simulink model "AI_Drivers"  (R2020b)
settings: Solver=VariableStepAuto  StartTime=0.0  StopTime=10.0  RelTol=1e-3
undefined symbols (not defined in the file): DiscIntNeverNeededParam
libraries: simulink x7, rllib x2, deeplib x1
(part 1 of 2)
settings Model: Creator=wenka  LastModifiedBy=wenka

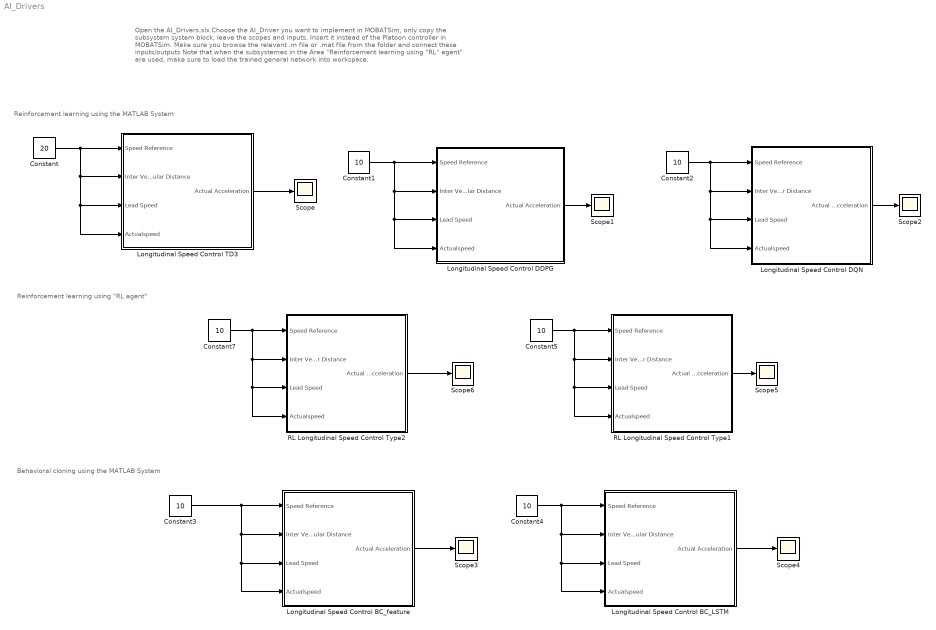
== system AI_Drivers ==
  note: Reinforcement learning using the MATLAB System
  note: Open the AI_Drivers.slx
      | Choose the AI_Driver you want to implement in MOBATSim, only copy the subsystem system block, leave the scopes and inputs.
      | Insert it instead of the Platoon controller in MOBATSim.
      | Make sure you browse the relevant .m file or .mat file from the folder and connect these inputs/outputs
      | Note that when the subsystemes in the Area "Reinforcement learning using "RL" agent" are used, make sure to load the trained general network into workspace.
  note: Behavioral cloning using the MATLAB System
  note: Reinforcement learning using "RL agent"
  Constant : Constant  Value=20  SampleTime=-1
  Constant{1..5,7} (6 alike) : Constant  Value=10  SampleTime=-1
  Longitudinal Speed Control BC_LSTM : Subsystem  mask{Ts=0.01, D_default=25, t_gap=2}
      mask prompts: Ts "Simulink:blkprm_prompts:AllSrcBlksSampleTime"; D_default "Default space"; t_gap "Time gap"
      mask TypeOptions Ts: RL Longitudinal Speed Control/Constant/SampleTime
      mask TypeOptions D_default: Subsystem/Subsystem1/Default Spacing/Value
      mask TypeOptions t_gap: Subsystem/Subsystem1/Time Gap/Value
      mask DialogControl Ts Prompt: Sample time:
  Longitudinal Speed Control BC_feature : Subsystem  mask{Ts=0.01, D_default=25, t_gap=2}
      mask prompts: Ts "Simulink:blkprm_prompts:AllSrcBlksSampleTime"; D_default "Default space"; t_gap "Time gap"
      mask TypeOptions Ts: RL Longitudinal Speed Control/Constant/SampleTime
      mask TypeOptions D_default: Subsystem/Subsystem1/Default Spacing/Value
      mask TypeOptions t_gap: Subsystem/Subsystem1/Time Gap/Value
      mask DialogControl Ts Prompt: Sample time:
  Longitudinal Speed Control DDPG : Subsystem  mask{Ts=0.01, D_default=25, t_gap=1.6}
      mask prompts: Ts "Simulink:blkprm_prompts:AllSrcBlksSampleTime"; D_default "Default space"; t_gap "Time gap"
      mask TypeOptions Ts: RL Longitudinal Speed Control/Constant/SampleTime
      mask TypeOptions D_default: Subsystem/Subsystem1/Default Spacing/Value
      mask TypeOptions t_gap: Subsystem/Subsystem1/Time Gap/Value
      mask DialogControl Ts Prompt: Sample time:
  Longitudinal Speed Control DQN : Subsystem  mask{Ts=0.01, D_default=25, t_gap=1.6}
      mask prompts: Ts "Simulink:blkprm_prompts:AllSrcBlksSampleTime"; D_default "Default space"; t_gap "Time gap"
      mask TypeOptions Ts: RL Longitudinal Speed Control/Constant/SampleTime
      mask TypeOptions D_default: Subsystem/Subsystem1/Default Spacing/Value
      mask TypeOptions t_gap: Subsystem/Subsystem1/Time Gap/Value
      mask DialogControl Ts Prompt: Sample time:
  Longitudinal Speed Control TD3 : Subsystem  mask{Ts=0.01, D_default=25, t_gap=1.6}
      mask prompts: Ts "Simulink:blkprm_prompts:AllSrcBlksSampleTime"; D_default "Default space"; t_gap "Time gap"
      mask TypeOptions Ts: RL Longitudinal Speed Control/Constant/SampleTime
      mask TypeOptions D_default: Subsystem/Subsystem1/Default Spacing/Value
      mask TypeOptions t_gap: Subsystem/Subsystem1/Time Gap/Value
      mask DialogControl Ts Prompt: Sample time:
  RL Longitudinal Speed Control Type1 : Subsystem  mask{Ts=0.01, D_default=25, t_gap=1.6}
      mask prompts: Ts "Simulink:blkprm_prompts:AllSrcBlksSampleTime"; D_default "Default space"; t_gap "Time gap"
      mask TypeOptions Ts: RL Longitudinal Speed Control/Constant/SampleTime
      mask TypeOptions D_default: Subsystem/Subsystem1/Default Spacing/Value
      mask TypeOptions t_gap: Subsystem/Subsystem1/Time Gap/Value
      mask DialogControl Ts Prompt: Sample time:
  RL Longitudinal Speed Control Type2 : Subsystem  mask{Ts=0.01, D_default=25, t_gap=1.6}
      mask prompts: Ts "Simulink:blkprm_prompts:AllSrcBlksSampleTime"; D_default "Default space"; t_gap "Time gap"
      mask TypeOptions Ts: RL Longitudinal Speed Control/Constant/SampleTime
      mask TypeOptions D_default: Subsystem/Subsystem1/Default Spacing/Value
      mask TypeOptions t_gap: Subsystem/Subsystem1/Time Gap/Value
      mask DialogControl Ts Prompt: Sample time:
  Scope{,1..6} (7 alike) : Scope
  wires:
  Constant/1 -> Longitudinal Speed Control TD3/3(Lead Speed), Longitudinal Speed Control TD3/4(Actualspeed), Longitudinal Speed Control TD3/2(Inter Vehicular Distance), Longitudinal Speed Control TD3/1(Speed Reference)
  Constant1/1 -> Longitudinal Speed Control DDPG/4(Actualspeed), Longitudinal Speed Control DDPG/3(Lead Speed), Longitudinal Speed Control DDPG/2(Inter Vehicular Distance), Longitudinal Speed Control DDPG/1(Speed Reference)
  Longitudinal Speed Control TD3/1(Actual Acceleration) -> Scope/1
  Longitudinal Speed Control DDPG/1(Actual Acceleration) -> Scope1/1
  Constant2/1 -> Longitudinal Speed Control DQN/3(Lead Speed), Longitudinal Speed Control DQN/4(Actualspeed), Longitudinal Speed Control DQN/2(Inter Vehicular Distance), Longitudinal Speed Control DQN/1(Speed Reference)
  Longitudinal Speed Control DQN/1(Actual Acceleration) -> Scope2/1
  Constant3/1 -> Longitudinal Speed Control BC_feature/4(Actualspeed), Longitudinal Speed Control BC_feature/3(Lead Speed), Longitudinal Speed Control BC_feature/2(Inter Vehicular Distance), Longitudinal Speed Control BC_feature/1(Speed Reference)
  Longitudinal Speed Control BC_feature/1(Actual Acceleration) -> Scope3/1
  Constant4/1 -> Longitudinal Speed Control BC_LSTM/2(Inter Vehicular Distance), Longitudinal Speed Control BC_LSTM/3(Lead Speed), Longitudinal Speed Control BC_LSTM/4(Actualspeed), Longitudinal Speed Control BC_LSTM/1(Speed Reference)
  Longitudinal Speed Control BC_LSTM/1(Actual Acceleration) -> Scope4/1
  Constant5/1 -> RL Longitudinal Speed Control Type1/1(Speed Reference), RL Longitudinal Speed Control Type1/2(Inter Vehicular Distance), RL Longitudinal Speed Control Type1/4(Actualspeed), RL Longitudinal Speed Control Type1/3(Lead Speed)
  RL Longitudinal Speed Control Type1/1(Actual Acceleration) -> Scope5/1
  Constant7/1 -> RL Longitudinal Speed Control Type2/1(Speed Reference), RL Longitudinal Speed Control Type2/2(Inter Vehicular Distance), RL Longitudinal Speed Control Type2/3(Lead Speed), RL Longitudinal Speed Control Type2/4(Actualspeed)
  RL Longitudinal Speed Control Type2/1(Actual Acceleration) -> Scope6/1

== system AI_Drivers/Longitudinal Speed Control BC_LSTM ==
  note: The block processes the states, rewards and status for training the agent
  note: Output
  note: Reference speed
  note: Speed of the
      | lead vehicle
  note: Distance to the
      | lead vehicle
  note: Input
  note: Actual speed
  Speed Reference : Inport
  Inter Vehicular Distance : Inport  Port=2
  Lead Speed : Inport  Port=3
  Actualspeed : Inport  Port=4
  LSTM_prediction : Subsystem
  Signal Processing for ACC : Subsystem
  Actual Acceleration : Outport  VectorParamsAs1DForOutWhenUnconnected=off
  wires:
  Lead Speed/1 -> Signal Processing for ACC/3(v_lead)
  LSTM_prediction/1(Predicted Acc) -> Actual Acceleration/1
  Speed Reference/1 -> Signal Processing for ACC/2(v_ref)
  Actualspeed/1 -> Signal Processing for ACC/1(v_ego)
  Inter Vehicular Distance/1 -> Signal Processing for ACC/4(d_rel)
  Signal Processing for ACC/1(obs) -> LSTM_prediction/1("dataTest ")

== system AI_Drivers/Longitudinal Speed Control BC_feature ==
  note: The block processes the states, rewards and status for training the agent
  note: Output
  note: Reference speed
  note: Speed of the
      | lead vehicle
  note: Distance to the
      | lead vehicle
  note: Input
  note: Actual speed
  Speed Reference : Inport
  Inter Vehicular Distance : Inport  Port=2
  Lead Speed : Inport  Port=3
  Actualspeed : Inport  Port=4
  MATLAB System : MATLABSystem  System=BC_feature  SimulateUsing=Interpreted execution
      mask Type: BC_feature
      mask Display:
      | disp('BC_feature');
      | port_label('input',1,'DataInput');
      | port_label('output',1,'predictedData');
  Signal Processing for ACC : Subsystem
  Actual Acceleration : Outport  VectorParamsAs1DForOutWhenUnconnected=off
  wires:
  Lead Speed/1 -> Signal Processing for ACC/3(v_lead)
  MATLAB System/1 -> Actual Acceleration/1  "Acc"
  Speed Reference/1 -> Signal Processing for ACC/2(v_ref)
  Actualspeed/1 -> Signal Processing for ACC/1(v_ego)
  Inter Vehicular Distance/1 -> Signal Processing for ACC/4(d_rel)
  Signal Processing for ACC/1(obs) -> MATLAB System/1

== system AI_Drivers/Longitudinal Speed Control DDPG ==
  note: The block processes the states, rewards and status for training the agent
  note: Output
  note: Reference speed
  note: Speed of the
      | lead vehicle
  note: Distance to the
      | lead vehicle
  note: Input
  note: Actual speed
  Speed Reference : Inport
  Inter Vehicular Distance : Inport  Port=2
  Lead Speed : Inport  Port=3
  Actualspeed : Inport  Port=4
  Data Type Conversion : DataTypeConversion  OutDataTypeStr=double
  MATLAB System : MATLABSystem  System=DDPG  SimulateUsing=Interpreted execution
      mask Type: DDPG
      mask Display:
      | disp('DDPG');
      | port_label('input',1,'Obs');
      | port_label('output',1,'predictedAcc');
  Signal Processing for ACC : Subsystem
  Actual Acceleration : Outport  VectorParamsAs1DForOutWhenUnconnected=off
  wires:
  Lead Speed/1 -> Signal Processing for ACC/3(v_lead)
  Speed Reference/1 -> Signal Processing for ACC/2(v_ref)
  Actualspeed/1 -> Signal Processing for ACC/1(v_ego)
  Inter Vehicular Distance/1 -> Signal Processing for ACC/4(d_rel)
  Signal Processing for ACC/1(obs) -> MATLAB System/1
  Data Type Conversion/1 -> Actual Acceleration/1
  MATLAB System/1 -> Data Type Conversion/1  "Acc"

== system AI_Drivers/Longitudinal Speed Control DQN ==
  note: Reference speed
  note: The block processes observations for training the agent
  note: Distance to the
      | lead vehicle
  note: Input
  note: Actual speed
  note: Speed of the
      | lead vehicle
  note: Output
  Speed Reference : Inport
  Inter Vehicular Distance : Inport  Port=2
  Lead Speed : Inport  Port=3
  Actualspeed : Inport  Port=4
  MATLAB System : MATLABSystem  System=DQN  SimulateUsing=Interpreted execution
      mask Type: DQN
      mask Display:
      | disp('DQN');
      | port_label('input',1,'Obs');
      | port_label('input',2,'Action');
      | port_label('output',1,'predictedAcc');
  Signal Processing for ACC : Subsystem
  Unit Delay : UnitDelay  InitialCondition=0.01  SampleTime=Ts  HasFrameUpgradeWarning=on
  Actual Acceleration : Outport  VectorParamsAs1DForOutWhenUnconnected=off
  wires:
  Inter Vehicular Distance/1 -> Signal Processing for ACC/4(d_rel)
  Actualspeed/1 -> Signal Processing for ACC/1(v_ego)
  Speed Reference/1 -> Signal Processing for ACC/2(v_ref)
  Lead Speed/1 -> Signal Processing for ACC/3(v_lead)
  MATLAB System/1 -> Unit Delay/1, Actual Acceleration/1
  Unit Delay/1 -> MATLAB System/2
  Signal Processing for ACC/1(obs) -> MATLAB System/1

== system AI_Drivers/Longitudinal Speed Control TD3 ==
  note: The block processes the states, rewards and status for training the agent
  note: Output
  note: Reference speed
  note: Speed of the
      | lead vehicle
  note: Distance to the
      | lead vehicle
  note: Input
  note: Actual speed
  Speed Reference : Inport
  Inter Vehicular Distance : Inport  Port=2
  Lead Speed : Inport  Port=3
  Actualspeed : Inport  Port=4
  MATLAB System : MATLABSystem  System=TD3  SimulateUsing=Interpreted execution
      mask Type: TD3
      mask Display:
      | disp('TD3');
      | port_label('input',1,'Obs');
      | port_label('output',1,'predictedAcc');
  Signal Processing for ACC : Subsystem
  Actual Acceleration : Outport  VectorParamsAs1DForOutWhenUnconnected=off
  wires:
  Lead Speed/1 -> Signal Processing for ACC/3(v_lead)
  MATLAB System/1 -> Actual Acceleration/1  "Acc"
  Speed Reference/1 -> Signal Processing for ACC/2(v_ref)
  Actualspeed/1 -> Signal Processing for ACC/1(v_ego)
  Inter Vehicular Distance/1 -> Signal Processing for ACC/4(d_rel)
  Signal Processing for ACC/1(obs) -> MATLAB System/1

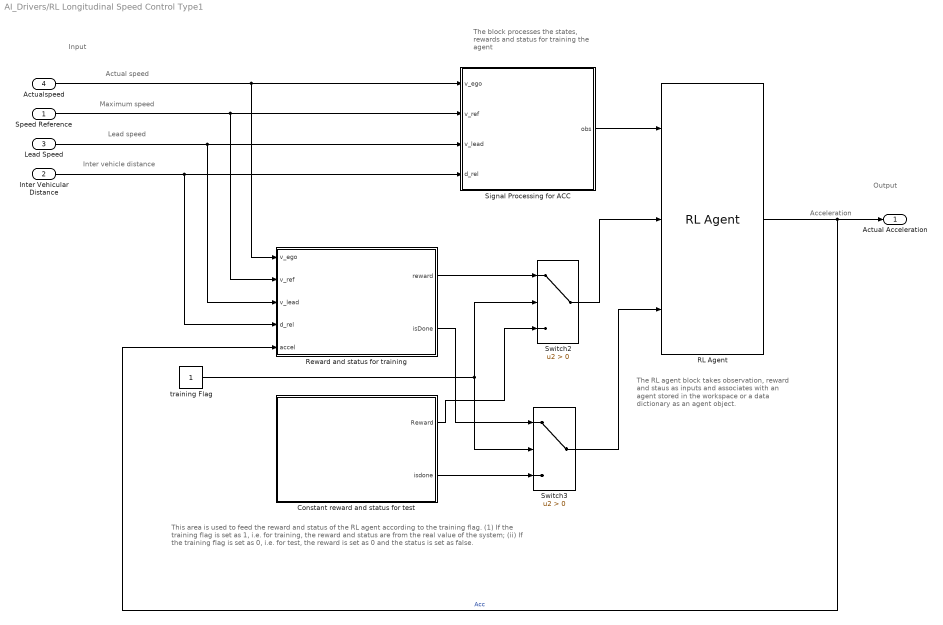
== system AI_Drivers/RL Longitudinal Speed Control Type1 ==
  note: Actual speed
  note: Acceleration
  note: Input
  note: Inter vehicle distance
  note: Lead speed
  note: Output
  note: The RL agent block takes observation, reward and staus as inputs and associates with an agent stored in the workspace or a data dictionary as an agent object.
  note: The block processes the states, rewards and status for training the agent
  note: Maximum speed
  note: This area is used to feed the reward and status of the RL agent according to the training flag.
      | (1) If the training flag is set as 1, i.e. for training, the reward and status are from the real value of the system;
      | (ii) If the training flag is set as 0, i.e. for test, the reward is set as 0 and the status is set as false.
  Speed Reference : Inport
  Inter Vehicular Distance : Inport  Port=2
  Lead Speed : Inport  Port=3
  Actualspeed : Inport  Port=4
  Constant reward and status for test : Subsystem
  RL Agent : rllib/RL Agent  Agent=agent  ProvideReward=on  ProvideIsDone=on  ProvideCumRwd=off  TreatAsDirectFeedthrough=on  CollectLoggedSignals=on  CollectModelStates=on
  Reward and status for training : Subsystem
  Signal Processing for ACC : Subsystem
  Switch2 : Switch  Criteria=u2 > Threshold
  Switch3 : Switch  Criteria=u2 > Threshold
  training Flag : Constant
  Actual Acceleration : Outport  VectorParamsAs1DForOutWhenUnconnected=off
  wires:
  Signal Processing for ACC/1(obs) -> RL Agent/1
  Actualspeed/1 -> Reward and status for training/1(v_ego), Signal Processing for ACC/1(v_ego)
  Speed Reference/1 -> Reward and status for training/2(v_ref), Signal Processing for ACC/2(v_ref)
  Lead Speed/1 -> Reward and status for training/3(v_lead), Signal Processing for ACC/3(v_lead)
  Inter Vehicular Distance/1 -> Reward and status for training/4(d_rel), Signal Processing for ACC/4(d_rel)
  Constant reward and status for test/2(isdone) -> Switch3/3
  training Flag/1 -> Switch2/2, Switch3/2
  Reward and status for training/1(reward) -> Switch2/1
  RL Agent/1 -> Reward and status for training/5(accel), Actual Acceleration/1  "Acc"
  Reward and status for training/2(isDone) -> Switch3/1
  Switch3/1 -> RL Agent/3
  Switch2/1 -> RL Agent/2
  Constant reward and status for test/1(Reward) -> Switch2/3

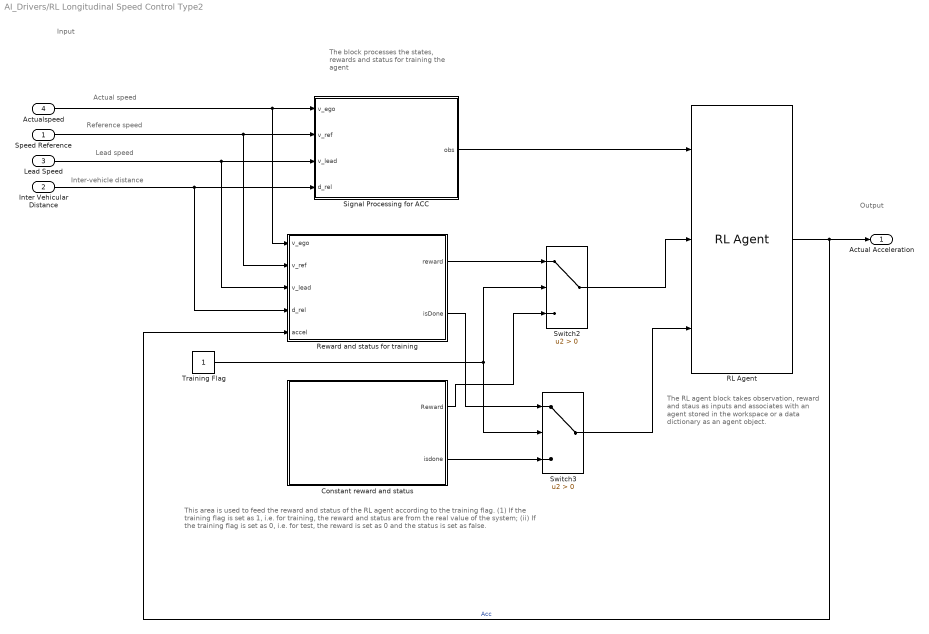
== system AI_Drivers/RL Longitudinal Speed Control Type2 ==
  note: Actual speed
  note: Input
  note: Reference speed
  note: Lead speed
  note: Output
  note: The block processes the states, rewards and status for training the agent
  note: The RL agent block takes observation, reward and staus as inputs and associates with an agent stored in the workspace or a data dictionary as an agent object.
  note: This area is used to feed the reward and status of the RL agent according to the training flag.
      | (1) If the training flag is set as 1, i.e. for training, the reward and status are from the real value of the system;
      | (ii) If the training flag is set as 0, i.e. for test, the reward is set as 0 and the status is set as false.
  note: Inter-vehicle distance
  Speed Reference : Inport
  Inter Vehicular Distance : Inport  Port=2
  Lead Speed : Inport  Port=3
  Actualspeed : Inport  Port=4
  Constant reward and status : Subsystem
  RL Agent : rllib/RL Agent  Agent=agent  ProvideReward=on  ProvideIsDone=on  ProvideCumRwd=off  TreatAsDirectFeedthrough=on  CollectLoggedSignals=on  CollectModelStates=on
  Reward and status for training : Subsystem
  Signal Processing for ACC : Subsystem
  Switch2 : Switch  Criteria=u2 > Threshold
  Switch3 : Switch  Criteria=u2 > Threshold
  Training Flag : Constant
  Actual Acceleration : Outport  VectorParamsAs1DForOutWhenUnconnected=off
  wires:
  Lead Speed/1 -> Reward and status for training/3(v_lead), Signal Processing for ACC/3(v_lead)
  Actualspeed/1 -> Reward and status for training/1(v_ego), Signal Processing for ACC/1(v_ego)
  Training Flag/1 -> Switch2/2, Switch3/2
  Constant reward and status/2(isdone) -> Switch3/3
  Reward and status for training/1(reward) -> Switch2/1
  Signal Processing for ACC/1(obs) -> RL Agent/1
  Reward and status for training/2(isDone) -> Switch3/1
  Switch3/1 -> RL Agent/3
  Switch2/1 -> RL Agent/2
  Constant reward and status/1(Reward) -> Switch2/3
  RL Agent/1 -> Reward and status for training/5(accel), Actual Acceleration/1  "Acc"
  Inter Vehicular Distance/1 -> Reward and status for training/4(d_rel), Signal Processing for ACC/4(d_rel)
  Speed Reference/1 -> Reward and status for training/2(v_ref), Signal Processing for ACC/2(v_ref)

== system AI_Drivers/Longitudinal Speed Control BC_LSTM/LSTM_prediction ==
  note: The Predict block predicts responses for the data at the input by using the trained network specified through the block parameter.
  note: This block normalizes the training predictors to have zero mean and unit variance
  "dataTest " : Inport
  MATLAB Function : MATLAB Function  TreatAsAtomicUnit=on  SystemSampleTime=Ts
  Mu File : FromFile  FileName=LSTM_mu.mat  SampleTime=0
  Predictor : deeplib/Predict  Network=Network from MAT-file  NetworkFunction=squeezenet  NetworkFilePath=C:\Users\wenka\OneDrive\Documents\GitHub\MOBATSim\AI_Drivers\BC_LSTM\BiLSTMnet.mat  MiniBatchSize=1  InputDataFormats={ '', '' }  Predictions=on  Activations={}  ForceInterpretedSim=off  EnableDLNetwork=off
      settings: SourceProductBaseCode=NN
  Sig File : FromFile  FileName=LSTM_sig.mat  SampleTime=0
  Predicted Acc : Outport
  wires:
  Sig File/1 -> MATLAB Function/3(sigFile)
  Predictor/1 -> Predicted Acc/1
  MATLAB Function/1(dataTest) -> Predictor/1
  "dataTest "/1 -> MATLAB Function/1("dataTest ")
  Mu File/1 -> MATLAB Function/2(muFile)

== system AI_Drivers/Longitudinal Speed Control BC_LSTM/Signal Processing for ACC ==
  note: observation
  note: Input
  note: Relative distance
  note: Ego speed
  note: Lead speed
  note: Maximum speed
  note: This subsystem calculates
      | the safe distance
  note: Output
  note: This subsystem calculates
      | the error between the ego
      | speed and target speed
  note: Relative distance
  note: Ego speed
  note: Speed error
  note: Lead speed
  note: Safe distance
  v_ego : Inport
  v_ref : Inport  Port=2
  v_lead : Inport  Port=3
  d_rel : Inport  Port=4
  Calculates speed error : Subsystem
  Mux : Mux  Inputs=5
  Safe distance : Subsystem
  obs : Outport  VectorParamsAs1DForOutWhenUnconnected=off
  wires:
  v_ego/1 -> Mux/5, Calculates speed error/3(v_ego), Safe distance/2(v_ego)
  d_rel/1 -> Mux/2, Safe distance/1(relative distance)
  Mux/1 -> obs/1
  Safe distance/2(Distance error) -> Calculates speed error/2(d_err)
  v_lead/1 -> Calculates speed error/1(v_lead), Mux/1
  v_ref/1 -> Calculates speed error/4(v_set)
  Safe distance/1(Safe distance) -> Mux/3
  Calculates speed error/1(v_err) -> Mux/4

== system AI_Drivers/Longitudinal Speed Control BC_feature/Signal Processing for ACC ==
  note: observation
  note: Input
  note: Relative distance
  note: Ego speed
  note: Lead speed
  note: Maximum speed
  note: This subsystem calculates
      | the safe distance
  note: Output
  note: This subsystem calculates
      | the error between the ego
      | speed and target speed
  note: Relative distance
  note: Ego speed
  note: Speed error
  note: Lead speed
  note: Safe distance
  v_ego : Inport
  v_ref : Inport  Port=2
  v_lead : Inport  Port=3
  d_rel : Inport  Port=4
  Calculates speed error : Subsystem
  Mux : Mux  Inputs=5
  Safe distance : Subsystem
  obs : Outport  VectorParamsAs1DForOutWhenUnconnected=off
  wires:
  v_ego/1 -> Mux/5, Calculates speed error/3(v_ego), Safe distance/2(v_ego)
  d_rel/1 -> Mux/2, Safe distance/1(relative distance)
  Mux/1 -> obs/1
  Safe distance/2(Distance error) -> Calculates speed error/2(d_err)
  v_lead/1 -> Calculates speed error/1(v_lead), Mux/1
  v_ref/1 -> Calculates speed error/4(v_set)
  Safe distance/1(Safe distance) -> Mux/3
  Calculates speed error/1(v_err) -> Mux/4

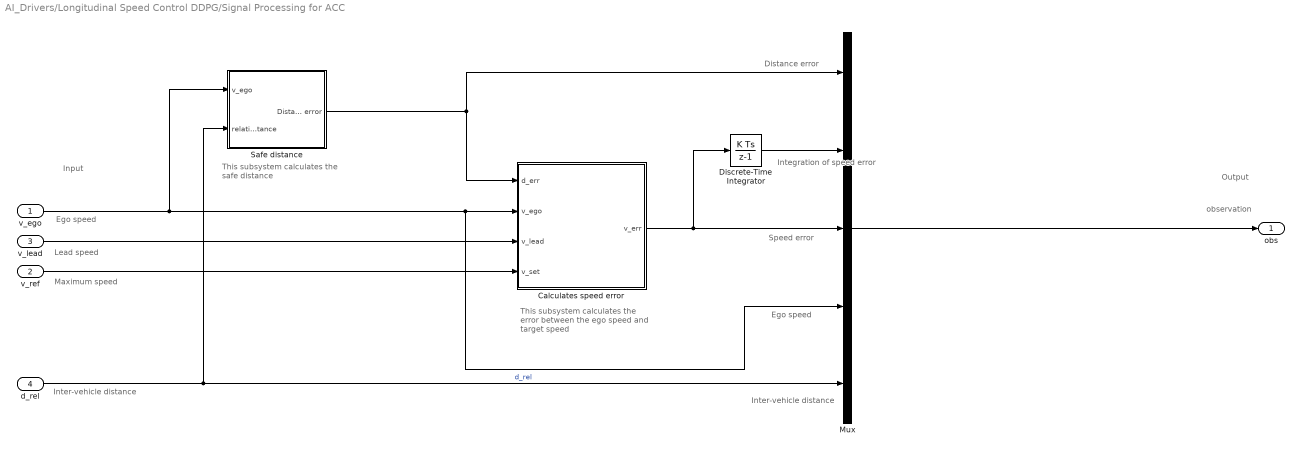
== system AI_Drivers/Longitudinal Speed Control DDPG/Signal Processing for ACC ==
  note: Distance error
  note: observation
  note: Input
  note: Inter-vehicle distance
  note: Ego speed
  note: Lead speed
  note: Maximum speed
  note: This subsystem calculates
      | the safe distance
  note: Output
  note: This subsystem calculates
      | the error between the ego
      | speed and target speed
  note: Inter-vehicle distance
  note: Ego speed
  note: Speed error
  note: Integration of
      | speed error
  v_ego : Inport
  v_ref : Inport  Port=2
  v_lead : Inport  Port=3
  d_rel : Inport  Port=4
  Calculates speed error : Subsystem
  Discrete-Time Integrator : DiscreteIntegrator  SampleTime=-1  ICPrevOutput=DiscIntNeverNeededParam  ICPrevScaledInput=DiscIntNeverNeededParam
  Mux : Mux  Inputs=5
  Safe distance : Subsystem
  obs : Outport  VectorParamsAs1DForOutWhenUnconnected=off
  wires:
  v_ego/1 -> Safe distance/1(v_ego), Calculates speed error/2(v_ego), Mux/4
  d_rel/1 -> Mux/5, Safe distance/2(relative distance)  "d_rel"
  Discrete-Time Integrator/1 -> Mux/2
  Safe distance/1(Distance error) -> Calculates speed error/1(d_err), Mux/1
  Calculates speed error/1(v_err) -> Discrete-Time Integrator/1, Mux/3
  v_lead/1 -> Calculates speed error/3(v_lead)
  v_ref/1 -> Calculates speed error/4(v_set)
  Mux/1 -> obs/1

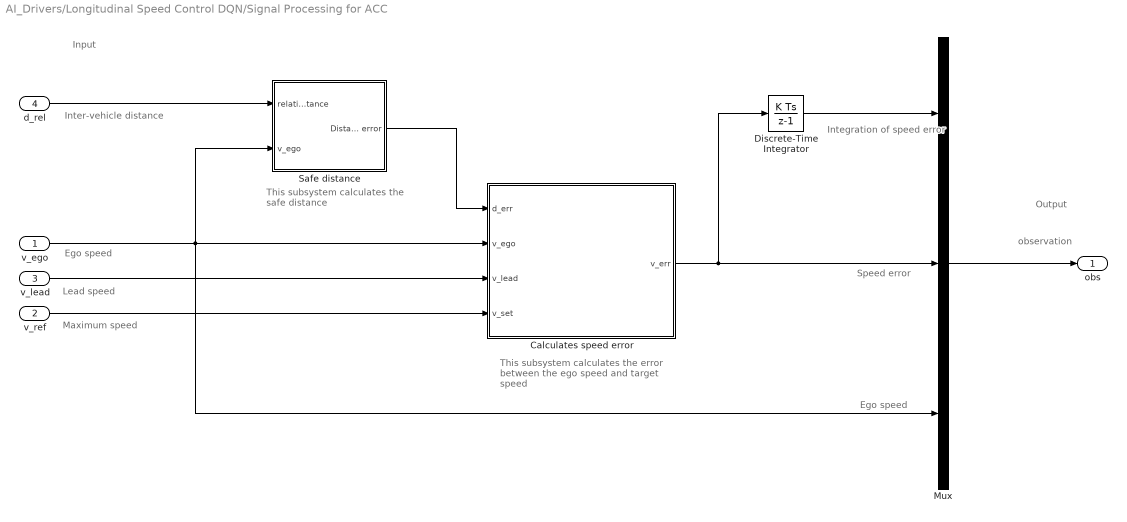
== system AI_Drivers/Longitudinal Speed Control DQN/Signal Processing for ACC ==
  note: observation
  note: Input
  note: Inter-vehicle distance
  note: Ego speed
  note: Lead speed
  note: Maximum speed
  note: This subsystem calculates
      | the safe distance
  note: Output
  note: This subsystem calculates
      | the error between the ego
      | speed and target speed
  note: Ego speed
  note: Speed error
  note: Integration of
      | speed error
  v_ego : Inport
  v_ref : Inport  Port=2
  v_lead : Inport  Port=3
  d_rel : Inport  Port=4
  Calculates speed error : Subsystem
  Discrete-Time Integrator : DiscreteIntegrator  SampleTime=-1  ICPrevOutput=DiscIntNeverNeededParam  ICPrevScaledInput=DiscIntNeverNeededParam
  Mux : Mux  Inputs=3
  Safe distance : Subsystem
  obs : Outport  VectorParamsAs1DForOutWhenUnconnected=off
  wires:
  v_ego/1 -> Mux/3, Safe distance/2(v_ego), Calculates speed error/2(v_ego)
  d_rel/1 -> Safe distance/1(relative distance)
  Safe distance/1(Distance error) -> Calculates speed error/1(d_err)
  Calculates speed error/1(v_err) -> Discrete-Time Integrator/1, Mux/2
  v_lead/1 -> Calculates speed error/3(v_lead)
  v_ref/1 -> Calculates speed error/4(v_set)
  Mux/1 -> obs/1
  Discrete-Time Integrator/1 -> Mux/1

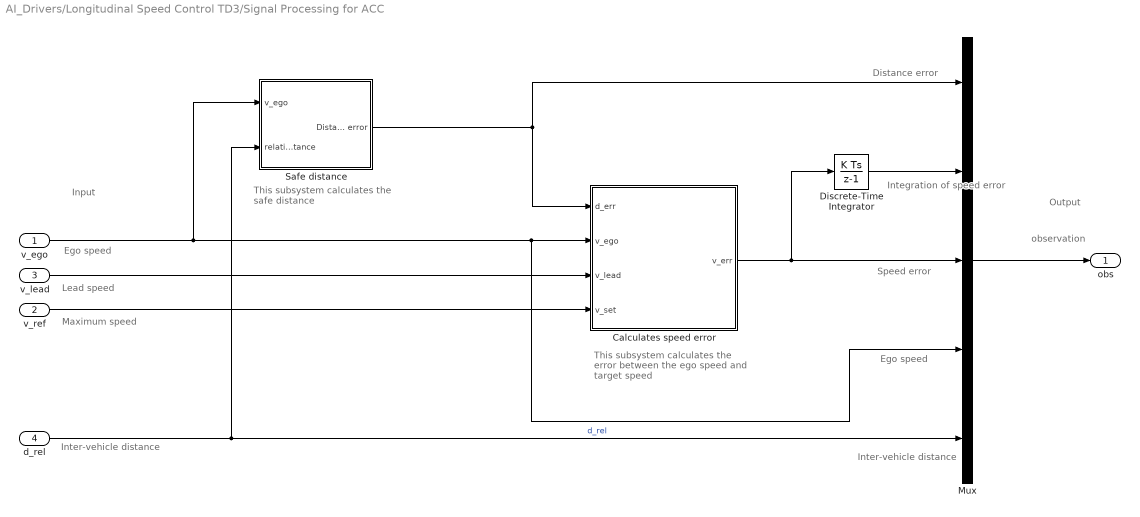
== system AI_Drivers/Longitudinal Speed Control TD3/Signal Processing for ACC ==
  note: Distance error
  note: observation
  note: Input
  note: Inter-vehicle distance
  note: Ego speed
  note: Lead speed
  note: Maximum speed
  note: This subsystem calculates
      | the safe distance
  note: Output
  note: This subsystem calculates
      | the error between the ego
      | speed and target speed
  note: Inter-vehicle distance
  note: Ego speed
  note: Speed error
  note: Integration of
      | speed error
  v_ego : Inport
  v_ref : Inport  Port=2
  v_lead : Inport  Port=3
  d_rel : Inport  Port=4
  Calculates speed error : Subsystem
  Discrete-Time Integrator : DiscreteIntegrator  SampleTime=-1  ICPrevOutput=DiscIntNeverNeededParam  ICPrevScaledInput=DiscIntNeverNeededParam
  Mux : Mux  Inputs=5
  Safe distance : Subsystem
  obs : Outport  VectorParamsAs1DForOutWhenUnconnected=off
  wires:
  v_ego/1 -> Safe distance/1(v_ego), Calculates speed error/2(v_ego), Mux/4
  d_rel/1 -> Mux/5, Safe distance/2(relative distance)  "d_rel"
  Discrete-Time Integrator/1 -> Mux/2
  Mux/1 -> obs/1
  Safe distance/1(Distance error) -> Calculates speed error/1(d_err), Mux/1
  Calculates speed error/1(v_err) -> Discrete-Time Integrator/1, Mux/3
  v_lead/1 -> Calculates speed error/3(v_lead)
  v_ref/1 -> Calculates speed error/4(v_set)

== system AI_Drivers/RL Longitudinal Speed Control Type1/Constant reward and status for test ==
  Cast To Boolean : DataTypeConversion  OutDataTypeStr=boolean
  Constant : Constant  Value=0  SampleTime=-1
  Reward : Outport
  isdone : Outport  Port=2
  wires:
  Cast To Boolean/1 -> isdone/1
  Constant/1 -> Cast To Boolean/1, Reward/1

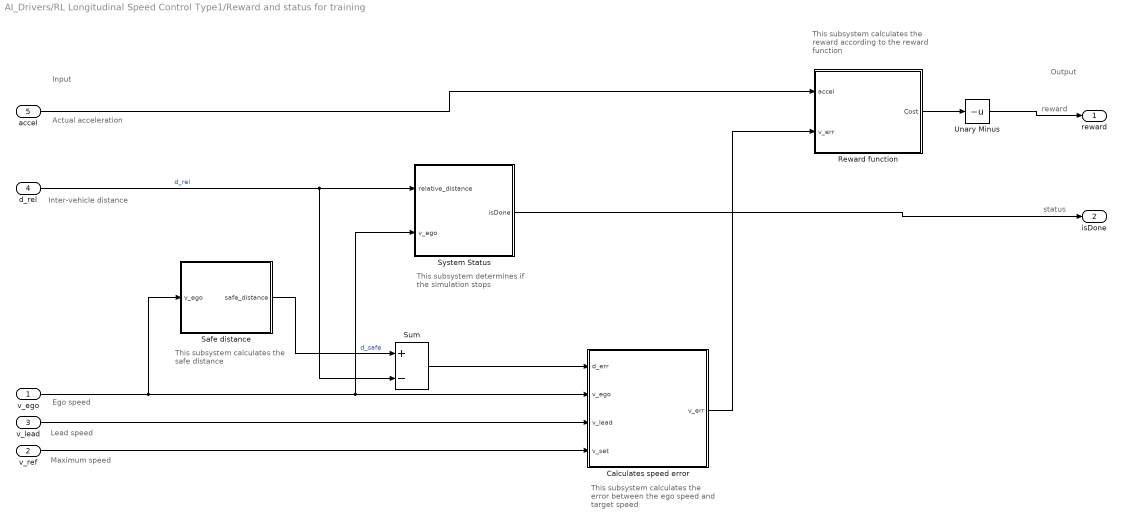
== system AI_Drivers/RL Longitudinal Speed Control Type1/Reward and status for training ==
  note: Input
  note: Actual acceleration
  note: reward
  note: Lead speed
  note: This subsystem determines
      | if the simulation stops
  note: Maximum speed
  note: Inter-vehicle distance
  note: This subsystem calculates
      | the safe distance
  note: Ego speed
  note: Output
  note: status
  note: This subsystem calculates
      | the reward according to the reward function
  note: This subsystem calculates
      | the error between the ego
      | speed and target speed
  v_ego : Inport
  v_ref : Inport  Port=2
  v_lead : Inport  Port=3
  d_rel : Inport  Port=4
  accel : Inport  Port=5
  Calculates speed error : Subsystem
  Reward function : Subsystem
  Safe distance : Subsystem
  Sum : Sum  Inputs=+-
  System Status : Subsystem
  Unary Minus : UnaryMinus
  reward : Outport  VectorParamsAs1DForOutWhenUnconnected=off
  isDone : Outport  Port=2  VectorParamsAs1DForOutWhenUnconnected=off
  wires:
  Safe distance/1(safe_distance) -> Sum/1  "d_safe"
  Reward function/1(Cost) -> Unary Minus/1
  v_lead/1 -> Calculates speed error/3(v_lead)
  v_ref/1 -> Calculates speed error/4(v_set)
  Calculates speed error/1(v_err) -> Reward function/2(v_err)
  accel/1 -> Reward function/1(accel)
  Sum/1 -> Calculates speed error/1(d_err)
  v_ego/1 -> Safe distance/1(v_ego), Calculates speed error/2(v_ego), System Status/2(v_ego)
  d_rel/1 -> Sum/2, System Status/1(relative_distance)  "d_rel"
  Unary Minus/1 -> reward/1
  System Status/1(isDone) -> isDone/1

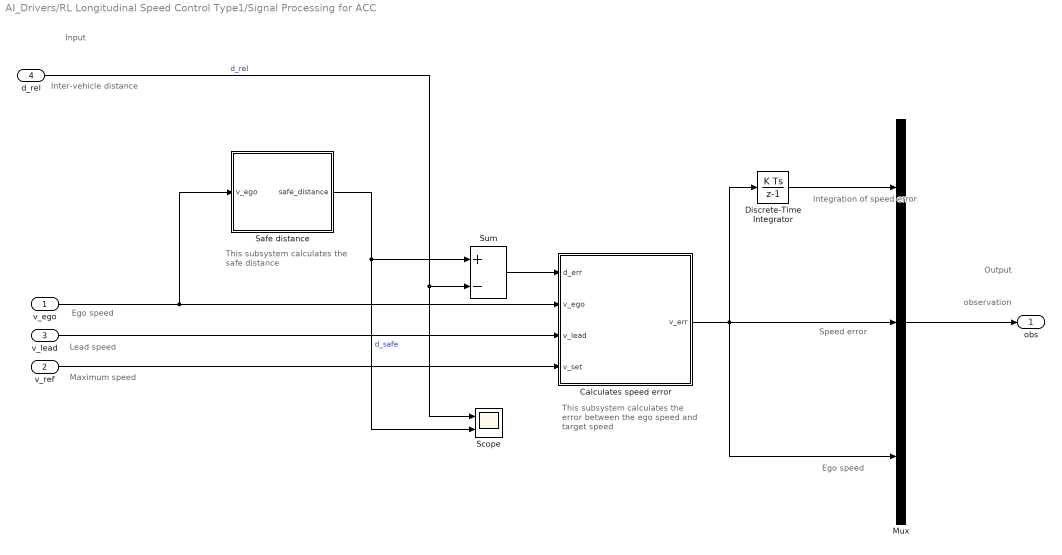
== system AI_Drivers/RL Longitudinal Speed Control Type1/Signal Processing for ACC ==
  note: observation
  note: Input
  note: Inter-vehicle distance
  note: Ego speed
  note: Lead speed
  note: Maximum speed
  note: This subsystem calculates
      | the safe distance
  note: Output
  note: This subsystem calculates
      | the error between the ego
      | speed and target speed
  note: Ego speed
  note: Speed error
  note: Integration of
      | speed error
  v_ego : Inport
  v_ref : Inport  Port=2
  v_lead : Inport  Port=3
  d_rel : Inport  Port=4
  Calculates speed error : Subsystem
  Discrete-Time Integrator : DiscreteIntegrator  SampleTime=-1  ICPrevOutput=DiscIntNeverNeededParam  ICPrevScaledInput=DiscIntNeverNeededParam
  Mux : Mux  Inputs=3
  Safe distance : Subsystem
  Scope : Scope  NumInputPorts=2
  Sum : Sum  Inputs=+-
  obs : Outport  VectorParamsAs1DForOutWhenUnconnected=off
  wires:
  v_ego/1 -> Safe distance/1(v_ego), Calculates speed error/2(v_ego)
  d_rel/1 -> Scope/1, Sum/2  "d_rel"
  Mux/1 -> obs/1
  Safe distance/1(safe_distance) -> Scope/2, Sum/1  "d_safe"
  Sum/1 -> Calculates speed error/1(d_err)
  Calculates speed error/1(v_err) -> Mux/3, Mux/2, Discrete-Time Integrator/1
  v_lead/1 -> Calculates speed error/3(v_lead)
  v_ref/1 -> Calculates speed error/4(v_set)
  Discrete-Time Integrator/1 -> Mux/1

== system AI_Drivers/RL Longitudinal Speed Control Type2/Constant reward and status ==
  Cast To Boolean : DataTypeConversion  OutDataTypeStr=boolean
  Constant : Constant  Value=0  SampleTime=-1
  Reward : Outport
  isdone : Outport  Port=2
  wires:
  Cast To Boolean/1 -> isdone/1
  Constant/1 -> Cast To Boolean/1, Reward/1

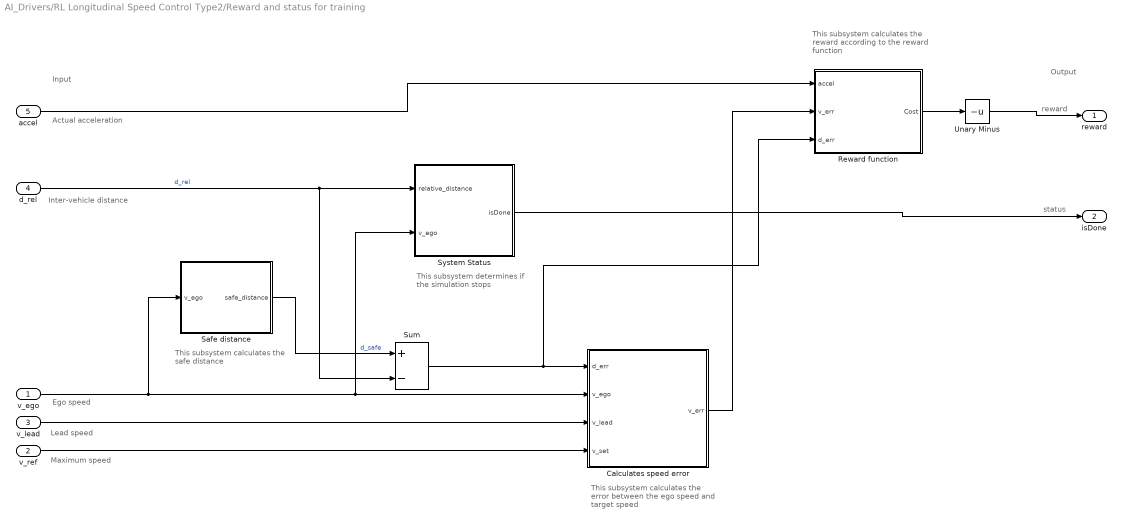
== system AI_Drivers/RL Longitudinal Speed Control Type2/Reward and status for training ==
  note: Input
  note: Actual acceleration
  note: reward
  note: Lead speed
  note: This subsystem determines
      | if the simulation stops
  note: Maximum speed
  note: Inter-vehicle distance
  note: This subsystem calculates
      | the safe distance
  note: Ego speed
  note: Output
  note: status
  note: This subsystem calculates
      | the reward according to the reward function
  note: This subsystem calculates
      | the error between the ego
      | speed and target speed
  v_ego : Inport
  v_ref : Inport  Port=2
  v_lead : Inport  Port=3
  d_rel : Inport  Port=4
  accel : Inport  Port=5
  Calculates speed error : Subsystem
  Reward function : Subsystem
  Safe distance : Subsystem
  Sum : Sum  Inputs=+-
  System Status : Subsystem
  Unary Minus : UnaryMinus
  reward : Outport  VectorParamsAs1DForOutWhenUnconnected=off
  isDone : Outport  Port=2  VectorParamsAs1DForOutWhenUnconnected=off
  wires:
  Safe distance/1(safe_distance) -> Sum/1  "d_safe"
  Reward function/1(Cost) -> Unary Minus/1
  v_lead/1 -> Calculates speed error/3(v_lead)
  v_ref/1 -> Calculates speed error/4(v_set)
  Calculates speed error/1(v_err) -> Reward function/2(v_err)
  accel/1 -> Reward function/1(accel)
  Sum/1 -> Calculates speed error/1(d_err), Reward function/3(d_err)
  v_ego/1 -> Safe distance/1(v_ego), Calculates speed error/2(v_ego), System Status/2(v_ego)
  d_rel/1 -> Sum/2, System Status/1(relative_distance)  "d_rel"
  Unary Minus/1 -> reward/1
  System Status/1(isDone) -> isDone/1

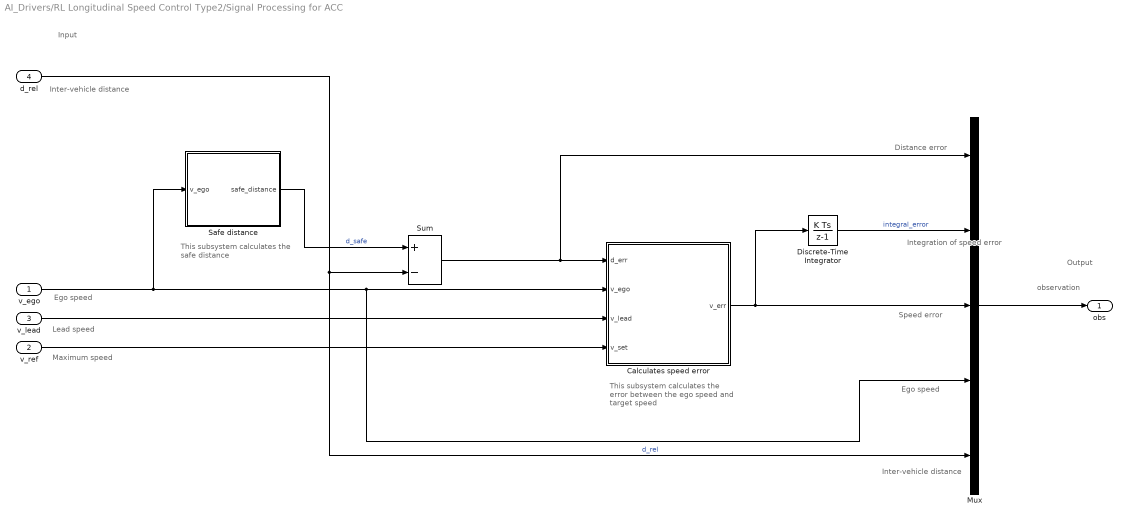
== system AI_Drivers/RL Longitudinal Speed Control Type2/Signal Processing for ACC ==
  note: Distance error
  note: observation
  note: Input
  note: Inter-vehicle distance
  note: Ego speed
  note: Lead speed
  note: Maximum speed
  note: This subsystem calculates
      | the safe distance
  note: Output
  note: This subsystem calculates
      | the error between the ego
      | speed and target speed
  note: Inter-vehicle distance
  note: Ego speed
  note: Speed error
  note: Integration of
      | speed error
  v_ego : Inport
  v_ref : Inport  Port=2
  v_lead : Inport  Port=3
  d_rel : Inport  Port=4
  Calculates speed error : Subsystem
  Discrete-Time Integrator : DiscreteIntegrator  SampleTime=-1  ICPrevOutput=DiscIntNeverNeededParam  ICPrevScaledInput=DiscIntNeverNeededParam
  Mux : Mux  Inputs=5
  Safe distance : Subsystem
  Sum : Sum  Inputs=+-
  obs : Outport  VectorParamsAs1DForOutWhenUnconnected=off
  wires:
  v_ego/1 -> Safe distance/1(v_ego), Calculates speed error/2(v_ego), Mux/4
  d_rel/1 -> Mux/5, Sum/2  "d_rel"
  Discrete-Time Integrator/1 -> Mux/2  "integral_error"
  Mux/1 -> obs/1
  Safe distance/1(safe_distance) -> Sum/1  "d_safe"
  Sum/1 -> Calculates speed error/1(d_err), Mux/1
  Calculates speed error/1(v_err) -> Discrete-Time Integrator/1, Mux/3
  v_lead/1 -> Calculates speed error/3(v_lead)
  v_ref/1 -> Calculates speed error/4(v_set)

== system AI_Drivers/Longitudinal Speed Control BC_LSTM/Signal Processing for ACC/Calculates speed error ==
  note: If the relative distance is less than the safe distance, the ego car tracks the minimum of the lead car velocity and driver-set velocity. In this manner, the ego car maintains some distance from the lead car. If the relative distance is greater than the safe distance, the ego car tracks the driver-set velocity.
  note: Lead speed
  note: e = V ref − V ego
  note: Error beween the
      | relative distance and
      | the safe distance
  note: Reference speed
  note: Ego vehicle speed
  note: Input
  note: Output
  v_lead : Inport
  d_err : Inport  Port=2
  v_ego : Inport  Port=3
  v_set : Inport  Port=4
  Min : MinMax  Inputs=2
  Sum1 : Sum  Inputs=+-
  Switch : Switch  Criteria=u2 > Threshold
  v_err : Outport  VectorParamsAs1DForOutWhenUnconnected=off
  wires:
  Sum1/1 -> v_err/1
  v_ego/1 -> Sum1/2
  Switch/1 -> Sum1/1  "v_ref"
  d_err/1 -> Switch/2
  v_set/1 -> Min/2, Switch/3
  Min/1 -> Switch/1
  v_lead/1 -> Min/1

== system AI_Drivers/Longitudinal Speed Control BC_LSTM/Signal Processing for ACC/Safe distance ==
  note: d safe =t gap ∗ V ego + D default .
  relative distance : Inport
  v_ego : Inport  Port=2
  Default Spacing : Constant  Value=D_default  SampleTime=0.01
  Product : Product
  Sum : Sum  Inputs=+-
  Sum2 : Sum
  Time Gap : Constant  Value=t_gap  SampleTime=Ts
  Safe distance : Outport  VectorParamsAs1DForOutWhenUnconnected=off
  Distance error : Outport  Port=2  VectorParamsAs1DForOutWhenUnconnected=off
  wires:
  Product/1 -> Sum2/2
  Time Gap/1 -> Product/2
  Default Spacing/1 -> Sum2/1
  v_ego/1 -> Product/1
  Sum2/1 -> Safe distance/1, Sum/1
  Sum/1 -> Distance error/1
  relative distance/1 -> Sum/2

== system AI_Drivers/Longitudinal Speed Control BC_feature/Signal Processing for ACC/Calculates speed error ==
  note: If the relative distance is less than the safe distance, the ego car tracks the minimum of the lead car velocity and driver-set velocity. In this manner, the ego car maintains some distance from the lead car. If the relative distance is greater than the safe distance, the ego car tracks the driver-set velocity.
  note: Lead speed
  note: e = V ref − V ego
  note: Error beween the
      | relative distance and
      | the safe distance
  note: Reference speed
  note: Ego vehicle speed
  note: Input
  note: Output
  v_lead : Inport
  d_err : Inport  Port=2
  v_ego : Inport  Port=3
  v_set : Inport  Port=4
  Min : MinMax  Inputs=2
  Sum1 : Sum  Inputs=+-
  Switch : Switch  Criteria=u2 > Threshold
  v_err : Outport  VectorParamsAs1DForOutWhenUnconnected=off
  wires:
  Sum1/1 -> v_err/1
  v_ego/1 -> Sum1/2
  Switch/1 -> Sum1/1  "v_ref"
  d_err/1 -> Switch/2
  v_set/1 -> Min/2, Switch/3
  Min/1 -> Switch/1
  v_lead/1 -> Min/1

== system AI_Drivers/Longitudinal Speed Control BC_feature/Signal Processing for ACC/Safe distance ==
  note: d safe =t gap ∗ V ego + D default .
  relative distance : Inport
  v_ego : Inport  Port=2
  Default Spacing : Constant  Value=D_default  SampleTime=0.01
  Product : Product
  Sum : Sum  Inputs=+-
  Sum2 : Sum
  Time Gap : Constant  Value=t_gap  SampleTime=Ts
  Safe distance : Outport  VectorParamsAs1DForOutWhenUnconnected=off
  Distance error : Outport  Port=2  VectorParamsAs1DForOutWhenUnconnected=off
  wires:
  Product/1 -> Sum2/2
  Time Gap/1 -> Product/2
  Default Spacing/1 -> Sum2/1
  v_ego/1 -> Product/1
  Sum2/1 -> Safe distance/1, Sum/1
  Sum/1 -> Distance error/1
  relative distance/1 -> Sum/2

== system AI_Drivers/Longitudinal Speed Control DDPG/Signal Processing for ACC/Calculates speed error ==
  note: If the relative distance is less than the safe distance, the ego car tracks the minimum of the lead car velocity and driver-set velocity. In this manner, the ego car maintains some distance from the lead car. If the relative distance is greater than the safe distance, the ego car tracks the driver-set velocity.
  note: Lead speed
  note: e = V ref − V ego
  note: Error beween the
      | relative distance and
      | the safe distance
  note: Reference speed
  note: Ego vehicle speed
  note: Input
  note: Output
  d_err : Inport
  v_ego : Inport  Port=2
  v_lead : Inport  Port=3
  v_set : Inport  Port=4
  Min : MinMax  Inputs=2
  Scope : Scope  NumInputPorts=3
  Sum1 : Sum  Inputs=+-
  Switch : Switch  Criteria=u2 > Threshold
  v_err : Outport  VectorParamsAs1DForOutWhenUnconnected=off
  wires:
  Sum1/1 -> v_err/1
  v_ego/1 -> Scope/2, Sum1/2  "v_ego"
  Switch/1 -> Scope/1, Sum1/1  "v_ref"
  d_err/1 -> Switch/2
  v_set/1 -> Min/2, Switch/3
  Min/1 -> Switch/1
  v_lead/1 -> Scope/3, Min/1  "v_lead"

== system AI_Drivers/Longitudinal Speed Control DDPG/Signal Processing for ACC/Safe distance ==
  note: d safe =t gap ∗ V ego + D default .
  v_ego : Inport
  relative distance : Inport  Port=2
  Default Spacing : Constant  Value=D_default  SampleTime=Ts
  Product : Product
  Scope : Scope  NumInputPorts=2
  Sum : Sum  Inputs=+-
  Sum2 : Sum
  Time Gap : Constant  Value=t_gap  SampleTime=Ts
  Distance error : Outport  VectorParamsAs1DForOutWhenUnconnected=off
  wires:
  Product/1 -> Sum2/2
  Time Gap/1 -> Product/2
  Default Spacing/1 -> Sum2/1
  v_ego/1 -> Product/1
  Sum2/1 -> Scope/1, Sum/1  "d_safe"
  Sum/1 -> Distance error/1
  relative distance/1 -> Scope/2, Sum/2  "d_rel"

== system AI_Drivers/Longitudinal Speed Control DQN/Signal Processing for ACC/Calculates speed error ==
  note: If the relative distance is less than the safe distance, the ego car tracks the minimum of the lead car velocity and driver-set velocity. In this manner, the ego car maintains some distance from the lead car. If the relative distance is greater than the safe distance, the ego car tracks the driver-set velocity.
  note: Lead speed
  note: e = V ref − V ego
  note: Error beween the
      | relative distance and
      | the safe distance
  note: Reference speed
  note: Ego vehicle speed
  note: Input
  note: Output
  d_err : Inport
  v_ego : Inport  Port=2
  v_lead : Inport  Port=3
  v_set : Inport  Port=4
  Min : MinMax  Inputs=2
  Scope : Scope  NumInputPorts=3
  Sum1 : Sum  Inputs=+-
  Switch : Switch  Criteria=u2 > Threshold
  v_err : Outport  VectorParamsAs1DForOutWhenUnconnected=off
  wires:
  Sum1/1 -> v_err/1
  v_ego/1 -> Scope/2, Sum1/2  "v_ego"
  Switch/1 -> Scope/1, Sum1/1  "v_ref"
  d_err/1 -> Switch/2
  v_set/1 -> Min/2, Switch/3
  Min/1 -> Switch/1
  v_lead/1 -> Scope/3, Min/1  "v_lead"

== system AI_Drivers/Longitudinal Speed Control DQN/Signal Processing for ACC/Safe distance ==
  note: d safe =t gap ∗ V ego + D default .
  relative distance : Inport
  v_ego : Inport  Port=2
  Default Spacing : Constant  Value=D_default  SampleTime=Ts
  Product : Product
  Scope : Scope  NumInputPorts=2
  Sum : Sum  Inputs=+-
  Sum2 : Sum
  Time Gap : Constant  Value=t_gap  SampleTime=Ts
  Distance error : Outport  VectorParamsAs1DForOutWhenUnconnected=off
  wires:
  Product/1 -> Sum2/2
  Time Gap/1 -> Product/2
  Default Spacing/1 -> Sum2/1
  v_ego/1 -> Product/1
  Sum2/1 -> Scope/1, Sum/1  "d_safe"
  Sum/1 -> Distance error/1
  relative distance/1 -> Scope/2, Sum/2  "d_rel"

== system AI_Drivers/Longitudinal Speed Control TD3/Signal Processing for ACC/Calculates speed error ==
  note: If the relative distance is less than the safe distance, the ego car tracks the minimum of the lead car velocity and driver-set velocity. In this manner, the ego car maintains some distance from the lead car. If the relative distance is greater than the safe distance, the ego car tracks the driver-set velocity.
  note: Lead speed
  note: e = V ref − V ego
  note: Error beween the
      | relative distance and
      | the safe distance
  note: Reference speed
  note: Ego vehicle speed
  note: Input
  note: Output
  d_err : Inport
  v_ego : Inport  Port=2
  v_lead : Inport  Port=3
  v_set : Inport  Port=4
  Min : MinMax  Inputs=2
  Sum1 : Sum  Inputs=+-
  Switch : Switch  Criteria=u2 > Threshold
  v_err : Outport  VectorParamsAs1DForOutWhenUnconnected=off
  wires:
  Sum1/1 -> v_err/1
  v_ego/1 -> Sum1/2
  Switch/1 -> Sum1/1  "v_ref"
  d_err/1 -> Switch/2
  v_set/1 -> Min/2, Switch/3
  Min/1 -> Switch/1
  v_lead/1 -> Min/1

== system AI_Drivers/Longitudinal Speed Control TD3/Signal Processing for ACC/Safe distance ==
  note: d safe =t gap ∗ V ego + D default .
  v_ego : Inport
  relative distance : Inport  Port=2
  Default Spacing : Constant  Value=D_default  SampleTime=0.01
  Product : Product
  Sum : Sum  Inputs=+-
  Sum2 : Sum
  Time Gap : Constant  Value=t_gap  SampleTime=Ts
  Distance error : Outport  VectorParamsAs1DForOutWhenUnconnected=off
  wires:
  Product/1 -> Sum2/2
  Time Gap/1 -> Product/2
  Default Spacing/1 -> Sum2/1
  v_ego/1 -> Product/1
  Sum2/1 -> Sum/1
  Sum/1 -> Distance error/1
  relative distance/1 -> Sum/2

== system AI_Drivers/RL Longitudinal Speed Control Type1/Reward and status for training/Calculates speed error ==
  note: If the relative distance is less than the safe distance, the ego car tracks the minimum of the lead car velocity and driver-set velocity. In this manner, the ego car maintains some distance from the lead car. If the relative distance is greater than the safe distance, the ego car tracks the driver-set velocity.
  note: Lead speed
  note: e = V ref − V ego
  note: Error beween the
      | relative distance and
      | the safe distance
  note: Reference speed
  note: Ego vehicle speed
  note: Input
  note: Output
  d_err : Inport
  v_ego : Inport  Port=2
  v_lead : Inport  Port=3
  v_set : Inport  Port=4
  Min : MinMax  Inputs=2
  Scope : Scope  NumInputPorts=3
  Sum1 : Sum  Inputs=+-
  Switch : Switch  Criteria=u2 > Threshold
  v_err : Outport  VectorParamsAs1DForOutWhenUnconnected=off
  wires:
  v_ego/1 -> Sum1/2, Scope/3  "v_ego"
  Switch/1 -> Scope/2, Sum1/1  "v_ref"
  d_err/1 -> Switch/2
  v_set/1 -> Min/2, Switch/3
  Min/1 -> Switch/1
  v_lead/1 -> Min/1
  Sum1/1 -> Scope/1, v_err/1  "v_err"

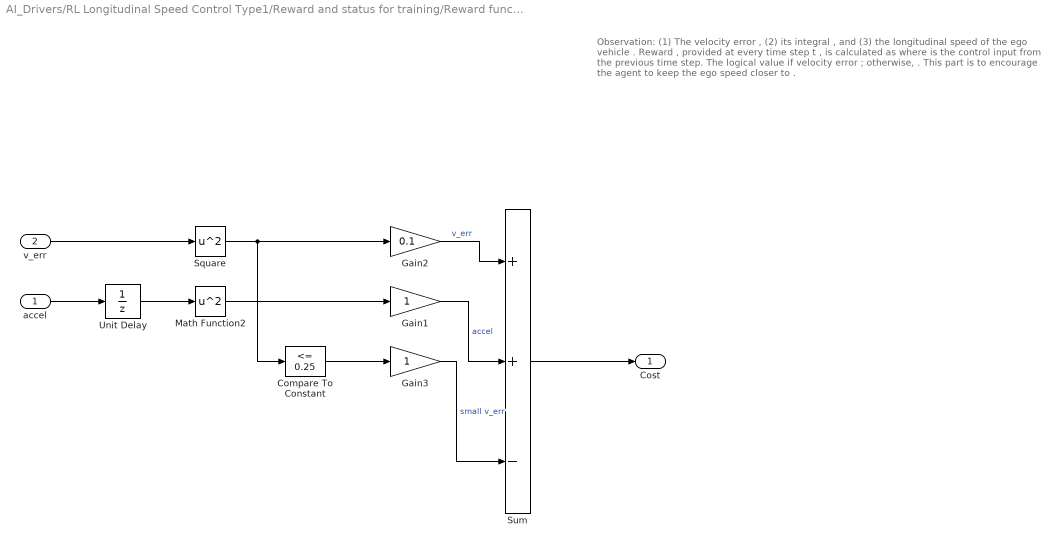
== system AI_Drivers/RL Longitudinal Speed Control Type1/Reward and status for training/Reward function ==
  note: Observation: (1) The velocity error , (2) its integral , and (3) the longitudinal speed of the ego vehicle .
      | Reward , provided at every time step t , is calculated as
      |
      | where is the control input from the previous time step. The logical value if velocity error ; otherwise, . This part is to encourage the agent to keep the ego speed closer to .
  accel : Inport
  v_err : Inport  Port=2
  Compare To Constant : simulink/Logic and Bit Operations/Compare To Constant  relop=<=  const=0.25  OutDataTypeStr=boolean
  Gain1 : Gain
  Gain2 : Gain  Gain=0.1
  Gain3 : Gain
  Math Function2 : Math  Operator=square  SignedPower=on  SaturateOnIntegerOverflow=on
  Square : Math  Operator=square  SignedPower=on  SaturateOnIntegerOverflow=on
  Sum : Sum  Inputs=++-
  Unit Delay : UnitDelay  SampleTime=-1  HasFrameUpgradeWarning=on
  Cost : Outport  VectorParamsAs1DForOutWhenUnconnected=off
  wires:
  v_err/1 -> Square/1
  Math Function2/1 -> Gain1/1
  accel/1 -> Unit Delay/1
  Square/1 -> Gain2/1, Compare To Constant/1
  Unit Delay/1 -> Math Function2/1
  Gain2/1 -> Sum/1  "v_err"
  Gain1/1 -> Sum/2  "accel"
  Compare To Constant/1 -> Gain3/1
  Gain3/1 -> Sum/3  "small v_err"
  Sum/1 -> Cost/1

== system AI_Drivers/RL Longitudinal Speed Control Type1/Reward and status for training/Safe distance ==
  note: d safe =t gap ∗ V ego + D default .
  v_ego : Inport
  Default Spacing : Constant  Value=D_default  SampleTime=Ts
  Product : Product
  Sum2 : Sum
  Time Gap : Constant  Value=t_gap  SampleTime=Ts
  safe_distance : Outport  VectorParamsAs1DForOutWhenUnconnected=off
  wires:
  Sum2/1 -> safe_distance/1
  Product/1 -> Sum2/2
  Time Gap/1 -> Product/2
  Default Spacing/1 -> Sum2/1
  v_ego/1 -> Product/1

== system AI_Drivers/RL Longitudinal Speed Control Type1/Reward and status for training/System Status ==
  note: If the distance to the lead vehicle is not positive or the speed is smaller than 0, then the status could be set as done.
  relative_distance : Inport
  v_ego : Inport  Port=2
  Logical Operator : Logic  Operator=OR  AllPortsSameDT=off  OutDataTypeStr=boolean
  Relative Distance : simulink/Logic and Bit Operations/Compare To Constant  relop=<  const=-1  OutDataTypeStr=boolean
  Velocity : simulink/Logic and Bit Operations/Compare To Constant  relop=<  const=0  OutDataTypeStr=boolean
  isDone : Outport  VectorParamsAs1DForOutWhenUnconnected=off
  wires:
  Velocity/1 -> Logical Operator/2
  Relative Distance/1 -> Logical Operator/1
  relative_distance/1 -> Relative Distance/1
  v_ego/1 -> Velocity/1
  Logical Operator/1 -> isDone/1

== system AI_Drivers/RL Longitudinal Speed Control Type1/Signal Processing for ACC/Calculates speed error ==
  note: If the relative distance is less than the safe distance, the ego car tracks the minimum of the lead car velocity and driver-set velocity. In this manner, the ego car maintains some distance from the lead car. If the relative distance is greater than the safe distance, the ego car tracks the driver-set velocity.
  note: Lead speed
  note: e = V ref − V ego
  note: Error beween the
      | relative distance and
      | the safe distance
  note: Reference speed
  note: Ego vehicle speed
  note: Input
  note: Output
  d_err : Inport
  v_ego : Inport  Port=2
  v_lead : Inport  Port=3
  v_set : Inport  Port=4
  Min : MinMax  Inputs=2
  Scope : Scope  NumInputPorts=3
  Sum1 : Sum  Inputs=+-
  Switch : Switch  Criteria=u2 > Threshold
  v_err : Outport  VectorParamsAs1DForOutWhenUnconnected=off
  wires:
  v_ego/1 -> Sum1/2, Scope/3  "v_ego"
  Switch/1 -> Scope/2, Sum1/1  "v_ref"
  d_err/1 -> Switch/2
  v_set/1 -> Min/2, Switch/3
  Min/1 -> Switch/1
  v_lead/1 -> Min/1
  Sum1/1 -> Scope/1, v_err/1  "v_err"

== system AI_Drivers/RL Longitudinal Speed Control Type1/Signal Processing for ACC/Safe distance ==
  note: d safe =t gap ∗ V ego + D default .
  v_ego : Inport
  Default Spacing : Constant  Value=D_default  SampleTime=Ts
  Product : Product
  Sum2 : Sum
  Time Gap : Constant  Value=t_gap  SampleTime=Ts
  safe_distance : Outport  VectorParamsAs1DForOutWhenUnconnected=off
  wires:
  Sum2/1 -> safe_distance/1
  Product/1 -> Sum2/2
  Time Gap/1 -> Product/2
  Default Spacing/1 -> Sum2/1
  v_ego/1 -> Product/1

== system AI_Drivers/RL Longitudinal Speed Control Type2/Reward and status for training/Calculates speed error ==
  note: If the relative distance is less than the safe distance, the ego car tracks the minimum of the lead car velocity and driver-set velocity. In this manner, the ego car maintains some distance from the lead car. If the relative distance is greater than the safe distance, the ego car tracks the driver-set velocity.
  note: Lead speed
  note: e = V ref − V ego
  note: Error beween the
      | relative distance and
      | the safe distance
  note: Reference speed
  note: Ego vehicle speed
  note: Input
  note: Output
  d_err : Inport
  v_ego : Inport  Port=2
  v_lead : Inport  Port=3
  v_set : Inport  Port=4
  Min : MinMax  Inputs=2
  Scope : Scope  NumInputPorts=3
  Sum1 : Sum  Inputs=+-
  Switch : Switch  Criteria=u2 > Threshold
  v_err : Outport  VectorParamsAs1DForOutWhenUnconnected=off
  wires:
  v_ego/1 -> Sum1/2, Scope/3  "v_ego"
  Switch/1 -> Scope/2, Sum1/1  "v_ref"
  d_err/1 -> Switch/2
  v_set/1 -> Min/2, Switch/3
  Min/1 -> Switch/1
  v_lead/1 -> Min/1
  Sum1/1 -> Scope/1, v_err/1  "v_err"

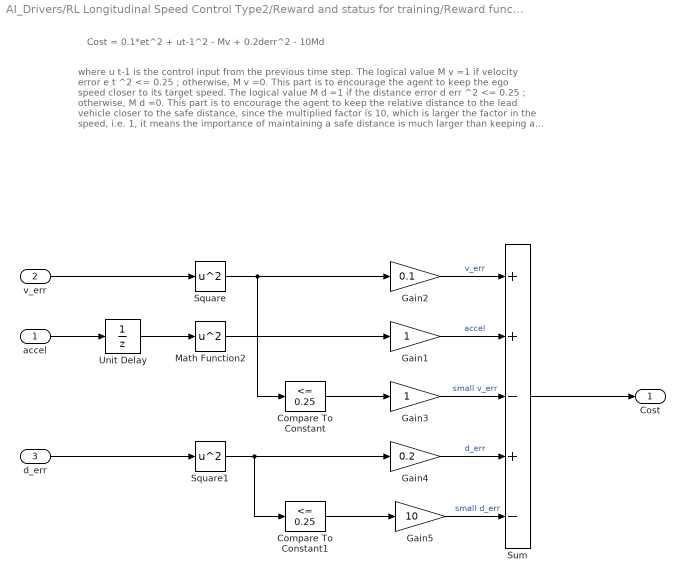
== system AI_Drivers/RL Longitudinal Speed Control Type2/Reward and status for training/Reward function ==
  note: Cost = 0.1*et^2 + ut-1^2 - Mv + 0.2derr^2 - 10Md
  note: where u t-1 is the control input from the previous time step. The logical value M v =1 if velocity error e t ^2 <= 0.25 ; otherwise, M v =0. This part is to encourage the agent to keep the ego speed closer to its target speed. The logical value M d =1 if the distance error d err ^2 <= 0.25 ; otherwise, M d =0. This part is to encourage the agent to keep the relative distance to the lead vehicle closer to the safe distance, since the multiplied factor is 10, which is larger the factor in the speed, i.e. 1, it means the importance of maintaining a safe distance is much larger than keeping a target speed. Cost = 0.1*et^2 + ut-1^2 - Mv + 0.2derr^2 - 10Md
  accel : Inport
  v_err : Inport  Port=2
  d_err : Inport  Port=3
  Compare To Constant : simulink/Logic and Bit Operations/Compare To Constant  relop=<=  const=0.25  OutDataTypeStr=boolean
  Compare To Constant1 : simulink/Logic and Bit Operations/Compare To Constant  relop=<=  const=0.25  OutDataTypeStr=boolean
  Gain1 : Gain
  Gain2 : Gain  Gain=0.1
  Gain3 : Gain
  Gain4 : Gain  Gain=0.2
  Gain5 : Gain  Gain=10
  Math Function2 : Math  Operator=square  SignedPower=on  SaturateOnIntegerOverflow=on
  Square : Math  Operator=square  SignedPower=on  SaturateOnIntegerOverflow=on
  Square1 : Math  Operator=square  SignedPower=on  SaturateOnIntegerOverflow=on
  Sum : Sum  Inputs=++-+-
  Unit Delay : UnitDelay  SampleTime=-1  HasFrameUpgradeWarning=on
  Cost : Outport  VectorParamsAs1DForOutWhenUnconnected=off
  wires:
  v_err/1 -> Square/1
  Math Function2/1 -> Gain1/1
  accel/1 -> Unit Delay/1
  Square/1 -> Gain2/1, Compare To Constant/1
  Unit Delay/1 -> Math Function2/1
  Gain2/1 -> Sum/1  "v_err"
  Gain1/1 -> Sum/2  "accel"
  Compare To Constant/1 -> Gain3/1
  Gain3/1 -> Sum/3  "small v_err"
  d_err/1 -> Square1/1
  Square1/1 -> Compare To Constant1/1, Gain4/1
  Gain4/1 -> Sum/4  "d_err"
  Compare To Constant1/1 -> Gain5/1
  Gain5/1 -> Sum/5  "small d_err"
  Sum/1 -> Cost/1

== system AI_Drivers/RL Longitudinal Speed Control Type2/Reward and status for training/Safe distance ==
  note: d safe =t gap ∗ V ego + D default .
  v_ego : Inport
  Default Spacing : Constant  Value=D_default  SampleTime=Ts
  Product : Product
  Sum2 : Sum
  Time Gap : Constant  Value=t_gap  SampleTime=Ts
  safe_distance : Outport  VectorParamsAs1DForOutWhenUnconnected=off
  wires:
  Sum2/1 -> safe_distance/1
  Product/1 -> Sum2/2
  Time Gap/1 -> Product/2
  Default Spacing/1 -> Sum2/1
  v_ego/1 -> Product/1

== system AI_Drivers/RL Longitudinal Speed Control Type2/Reward and status for training/System Status ==
  note: If the distance to the lead vehicle is not positive or the speed is smaller than 0, then the status could be set as done.
  relative_distance : Inport
  v_ego : Inport  Port=2
  Logical Operator : Logic  Operator=OR  AllPortsSameDT=off  OutDataTypeStr=boolean
  Relative Distance : simulink/Logic and Bit Operations/Compare To Constant  relop=<  const=-1  OutDataTypeStr=boolean
  Velocity : simulink/Logic and Bit Operations/Compare To Constant  relop=<  const=0  OutDataTypeStr=boolean
  isDone : Outport  VectorParamsAs1DForOutWhenUnconnected=off
  wires:
  Velocity/1 -> Logical Operator/2
  Relative Distance/1 -> Logical Operator/1
  relative_distance/1 -> Relative Distance/1
  v_ego/1 -> Velocity/1
  Logical Operator/1 -> isDone/1
